simulink model "untitled9"  (R2023b)
settings: Solver=FixedStepAuto  StartTime=0.0  StopTime=2.9  FixedStep=1e-5
values from neighbouring files (symbols this model uses):
  Global_Bx = reshape(Bx, [Nx, Ny, Nz])    [init_global_map2.m]
  Global_By = reshape(By, [Nx, Ny, Nz])    [init_global_map2.m]
  Global_Bz = reshape(Bz, [Nx, Ny, Nz])    [init_global_map2.m]
  N = Nx * Ny * Nz    (= 4080501)    [init_global_map2.m]
  x_glob_range = x_glob_range(:)    [init_global_map2.m]
  y_glob_range = y_glob_range(:)    [init_global_map2.m]
  z_glob_range = z_glob_range(:)    [init_global_map2.m]
undefined symbols (not defined in the file or in its folder): X, Y, Z
libraries: sm_lib x15, nesl_utility x6, sharedtransform x2, simulink x2
settings Model: Creator=germa  LastModifiedBy=germa

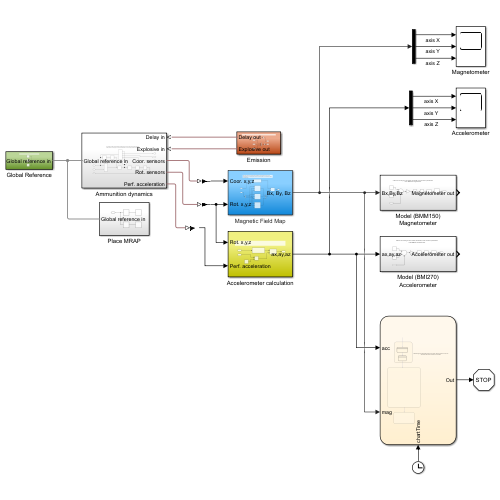
[thumbnail: Simulink's stored preview of the top-level diagram]
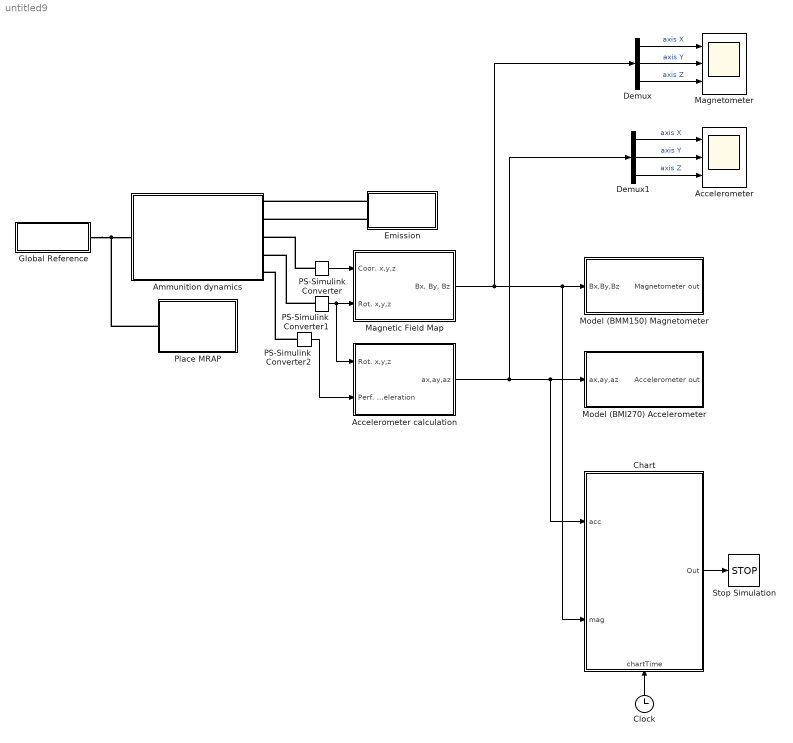
== system untitled9 ==
  Accelerometer : Scope  NumInputPorts=3
  Accelerometer calculation : Subsystem
  Ammunition dynamics : Subsystem
  Chart : Stateflow chart  TreatAsAtomicUnit=on
      settings: PortSchema="{\"entries\":[{\"content\":{\"sides\":[{\"content\":{\"connectorIds\":[\"In2\",\"In3\"]},\"type\":\"ConnectorPlacement.EquallySpacedRectSide\",\"uuid\":\"2f7f4fa5-e89a-4fc1-bed6-30d007998820\"},{\"content\":{\"connectorIds\":[\"Out1\"],\"side\":\"RIGHT\"},\"type\":\"ConnectorPlacement.EquallySpacedRectSide\",\"uuid\":\"4dcede0d-181a-4776-8973-11248acb9a50\"},{\"content\":{\"side\":\"TOP\"},\"type\":\"ConnectorPlacement.EquallySpacedRectSide\",\"uuid\":\"fd273f8e-25b4-48c5-b488-b01aba33f87d\"},{\"content\":{\"connectorIds\":[\"In1\"],\"side\":\"BOTTOM\"},\"type\":\"ConnectorPlacement.EquallySpacedRectSide\",\"uuid\":\"7dfac832-98a9-44a5-9739-cb7b49b62e5f\"}]},\"type\":\"ConnectorPlacement.EquallySpacedConnector\",\"uuid\":\"6be13ad6-9752-4a37-809e-31edad18d250\"}],\"packageUris\":[\"http://schema.mathworks.com/mf0/Connector/R2020b\"],\"version\":\"1.0\"}"
  Clock : Clock
  Demux : Demux  Outputs=3
  Demux1 : Demux  Outputs=3
  Emission : Subsystem
  Global Reference : Subsystem
  Magnetic Field Map : Subsystem
  Magnetometer : Scope  NumInputPorts=3
  Model (BMI270) Accelerometer : Subsystem
  Model (BMM150) Magnetometer : Subsystem
  PS-Simulink Converter : nesl_utility/PS-Simulink Converter  PhysicalDomain=network_engine_domain  SubClassName=ps_output  LeftPortType=input  RightPortType=output  PseudoPeriodic=off  Frequencies=[]  VectorFormat=inherit  Unit=inherit  AffineConversion=off
  PS-Simulink Converter1 : nesl_utility/PS-Simulink Converter  PhysicalDomain=network_engine_domain  SubClassName=ps_output  LeftPortType=input  RightPortType=output  PseudoPeriodic=off  Frequencies=[]  VectorFormat=inherit  Unit=inherit  AffineConversion=off
  PS-Simulink Converter2 : nesl_utility/PS-Simulink Converter  PhysicalDomain=network_engine_domain  SubClassName=ps_output  LeftPortType=input  RightPortType=output  PseudoPeriodic=off  Frequencies=[]  VectorFormat=inherit  Unit=inherit  AffineConversion=off
  Place MRAP : Subsystem
  Stop Simulation : Stop
  wires:
  PS-Simulink Converter/1 -> Magnetic Field Map/1(Coor. x,y,z)
  PS-Simulink Converter1/1 -> Accelerometer calculation/1(Rot. x,y,z), Magnetic Field Map/2(Rot. x,y,z)
  Demux/3 -> Magnetometer/3  "axis Z"
  Demux/2 -> Magnetometer/2  "axis Y"
  Demux/1 -> Magnetometer/1  "axis X"
  Magnetic Field Map/1("Bx, By, Bz") -> Demux/1, Chart/3(mag), Model (BMM150) Magnetometer/1(Bx,By,Bz)
  Demux1/3 -> Accelerometer/3  "axis Z"
  Demux1/1 -> Accelerometer/1  "axis X"
  Demux1/2 -> Accelerometer/2  "axis Y"
  PS-Simulink Converter2/1 -> Accelerometer calculation/2(Perf. acceleration)
  Accelerometer calculation/1(ax,ay,az) -> Chart/2(acc), Model (BMI270) Accelerometer/1(ax,ay,az), Demux1/1
  Clock/1 -> Chart/1(chartTime)
  Chart/1(Out) -> Stop Simulation/1
  connections:
  Emission/RConn2 -- Ammunition dynamics/RConn2
  Emission/RConn1 -- Ammunition dynamics/RConn1
  PS-Simulink Converter/LConn1 -- Ammunition dynamics/RConn3
  PS-Simulink Converter1/LConn1 -- Ammunition dynamics/RConn4
  Global Reference/LConn1 -- Place MRAP/LConn1 -- Ammunition dynamics/LConn1
  PS-Simulink Converter2/LConn1 -- Ammunition dynamics/RConn5

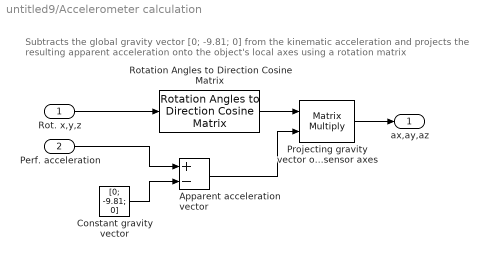
== system untitled9/Accelerometer calculation ==
  note: Subtracts the global gravity vector [0; -9.81; 0] from the kinematic acceleration and projects the resulting apparent acceleration onto the object's local axes using a rotation matrix
  Rot. x,y,z : Inport
  Perf. acceleration : Inport  Port=2
  Apparent acceleration vector : Sum  Inputs=+-
  Constant gravity vector : Constant  Value=[0; -9.81; 0]
  Projecting gravity vector onto sensor axes : Product  Multiplication=Matrix(*)
  Rotation Angles to Direction Cosine Matrix : sharedtransform/Rotation Angles to Direction Cosine Matrix  rotationOrder=XYZ  aMode=aMode
  ax,ay,az : Outport
  wires:
  Apparent acceleration vector/1 -> Projecting gravity vector onto sensor axes/2
  Perf. acceleration/1 -> Apparent acceleration vector/1
  Rot. x,y,z/1 -> Rotation Angles to Direction Cosine Matrix/1
  Rotation Angles to Direction Cosine Matrix/1 -> Projecting gravity vector onto sensor axes/1
  Constant gravity vector/1 -> Apparent acceleration vector/2
  Projecting gravity vector onto sensor axes/1 -> ax,ay,az/1

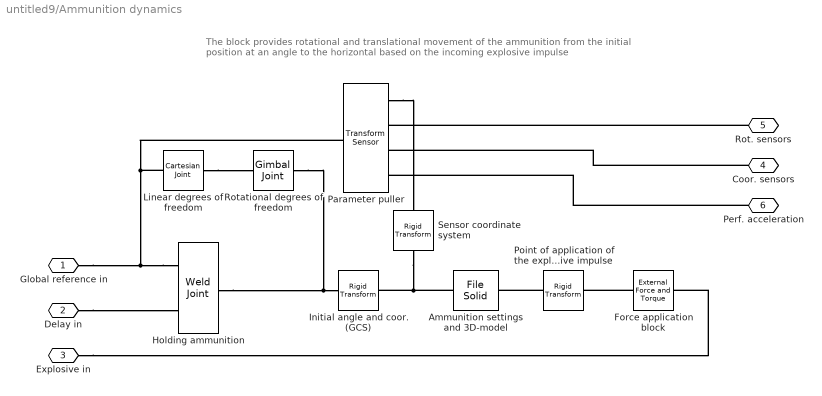
== system untitled9/Ammunition dynamics ==
  note: The block provides rotational and translational movement of the ammunition from the initial position at an angle to the horizontal based on the incoming explosive impulse
  "   Linear degrees of freedom" : sm_lib/Joints/Cartesian Joint  JointMode=Normal  SenseConstraintForce=off  SenseConstraintForceX=off  SenseConstraintForceY=off  SenseConstraintForceZ=off  SenseConstraintTorque=off  SenseConstraintTorqueX=off  SenseConstraintTorqueY=off  SenseConstraintTorqueZ=off  SenseTotalForce=off  SenseTotalForceX=off  SenseTotalForceY=off  SenseTotalForceZ=off  SenseTotalTorque=off  SenseTotalTorqueX=off  SenseTotalTorqueY=off  SenseTotalTorqueZ=off  CompositeWrenchDir=FollowerOnBase  CompositeWrenchFrame=BaseFrame  PxEquilibriumPosition=0  PxEquilibriumPositionUnits=m  PxSpringStiffness=0  PxSpringStiffnessUnits=N/m  PxDampingCoefficient=0  PxDampingCoefficientUnits=N/(m/s)  PxTorqueActuationMode=NoTorque  PxMotionActuationMode=ComputedMotion  PxSensePosition=off  PxSenseVelocity=off  PxSenseAcceleration=off  PxSenseTorqueForce=off  PxSenseLowerLimitTorqueForce=off  PxSenseUpperLimitTorqueForce=off  PxLowerLimitSpecify=off  PxLowerLimitBound=-1  PxLowerLimitBoundUnits=m  PxLowerLimitStiffness=1e6  PxLowerLimitStiffnessUnits=N/m  PxLowerLimitDamping=1e3  PxLowerLimitDampingUnits=N/(m/s)  PxLowerLimitTransitionRegionWidth=1e-4  PxLowerLimitTransitionRegionWidthUnits=m  PxUpperLimitSpecify=off  PxUpperLimitBound=1  PxUpperLimitBoundUnits=m  PxUpperLimitStiffness=1e6  PxUpperLimitStiffnessUnits=N/m  PxUpperLimitDamping=1e3  PxUpperLimitDampingUnits=N/(m/s)  PxUpperLimitTransitionRegionWidth=1e-4  PxUpperLimitTransitionRegionWidthUnits=m  PxPositionTargetSpecify=off  PxPositionTargetPriority=High  PxPositionTargetValue=0  PxPositionTargetValueUnits=m  PxVelocityTargetSpecify=off  PxVelocityTargetPriority=High  PxVelocityTargetValue=0  PxVelocityTargetValueUnits=m/s  PyEquilibriumPosition=0  PyEquilibriumPositionUnits=m  PySpringStiffness=0  PySpringStiffnessUnits=N/m  PyDampingCoefficient=0  PyDampingCoefficientUnits=N/(m/s)  PyTorqueActuationMode=NoTorque  PyMotionActuationMode=ComputedMotion  PySensePosition=off  PySenseVelocity=off  PySenseAcceleration=off  PySenseTorqueForce=off  PySenseLowerLimitTorqueForce=off  PySenseUpperLimitTorqueForce=off  PyLowerLimitSpecify=off  PyLowerLimitBound=-1  PyLowerLimitBoundUnits=m  PyLowerLimitStiffness=1e6  PyLowerLimitStiffnessUnits=N/m  PyLowerLimitDamping=1e3  PyLowerLimitDampingUnits=N/(m/s)  PyLowerLimitTransitionRegionWidth=1e-4  PyLowerLimitTransitionRegionWidthUnits=m  PyUpperLimitSpecify=off  PyUpperLimitBound=1  PyUpperLimitBoundUnits=m  PyUpperLimitStiffness=1e6  PyUpperLimitStiffnessUnits=N/m  PyUpperLimitDamping=1e3  PyUpperLimitDampingUnits=N/(m/s)  PyUpperLimitTransitionRegionWidth=1e-4  PyUpperLimitTransitionRegionWidthUnits=m  PyPositionTargetSpecify=off  PyPositionTargetPriority=High  PyPositionTargetValue=0  PyPositionTargetValueUnits=m  PyVelocityTargetSpecify=off  PyVelocityTargetPriority=High  PyVelocityTargetValue=0  PyVelocityTargetValueUnits=m/s  PzEquilibriumPosition=0  PzEquilibriumPositionUnits=m  PzSpringStiffness=0  PzSpringStiffnessUnits=N/m  PzDampingCoefficient=0  PzDampingCoefficientUnits=N/(m/s)  PzTorqueActuationMode=NoTorque  PzMotionActuationMode=ComputedMotion  PzSensePosition=off  PzSenseVelocity=off  PzSenseAcceleration=off  PzSenseTorqueForce=off  PzSenseLowerLimitTorqueForce=off  PzSenseUpperLimitTorqueForce=off  PzLowerLimitSpecify=off  PzLowerLimitBound=-1  PzLowerLimitBoundUnits=m  PzLowerLimitStiffness=1e6  PzLowerLimitStiffnessUnits=N/m  PzLowerLimitDamping=1e3  PzLowerLimitDampingUnits=N/(m/s)  PzLowerLimitTransitionRegionWidth=1e-4  PzLowerLimitTransitionRegionWidthUnits=m  PzUpperLimitSpecify=off  PzUpperLimitBound=1  PzUpperLimitBoundUnits=m  PzUpperLimitStiffness=1e6  PzUpperLimitStiffnessUnits=N/m  PzUpperLimitDamping=1e3  PzUpperLimitDampingUnits=N/(m/s)  PzUpperLimitTransitionRegionWidth=1e-4  PzUpperLimitTransitionRegionWidthUnits=m  PzPositionTargetSpecify=off  PzPositionTargetPriority=High  PzPositionTargetValue=0  PzPositionTargetValueUnits=m  PzVelocityTargetSpecify=off  PzVelocityTargetPriority=High  PzVelocityTargetValue=0  PzVelocityTargetValueUnits=m/s
  "  Rotational degrees of freedom" : sm_lib/Joints/Gimbal Joint  JointMode=Normal  SenseConstraintForce=off  SenseConstraintForceX=off  SenseConstraintForceY=off  SenseConstraintForceZ=off  SenseConstraintTorque=off  SenseConstraintTorqueX=off  SenseConstraintTorqueY=off  SenseConstraintTorqueZ=off  SenseTotalForce=off  SenseTotalForceX=off  SenseTotalForceY=off  SenseTotalForceZ=off  SenseTotalTorque=off  SenseTotalTorqueX=off  SenseTotalTorqueY=off  SenseTotalTorqueZ=off  CompositeWrenchDir=FollowerOnBase  CompositeWrenchFrame=BaseFrame  RxEquilibriumPosition=0  RxEquilibriumPositionUnits=deg  RxSpringStiffness=0  RxSpringStiffnessUnits=N*m/deg  RxDampingCoefficient=0  RxDampingCoefficientUnits=N*m/(deg/s)  RxTorqueActuationMode=NoTorque  RxMotionActuationMode=ComputedMotion  RxSensePosition=off  RxSenseVelocity=off  RxSenseAcceleration=off  RxSenseTorqueForce=off  RxSenseLowerLimitTorqueForce=off  RxSenseUpperLimitTorqueForce=off  RxLowerLimitSpecify=off  RxLowerLimitBound=-90  RxLowerLimitBoundUnits=deg  RxLowerLimitStiffness=1e4  RxLowerLimitStiffnessUnits=N*m/deg  RxLowerLimitDamping=10  RxLowerLimitDampingUnits=N*m/(deg/s)  RxLowerLimitTransitionRegionWidth=0.1  RxLowerLimitTransitionRegionWidthUnits=deg  RxUpperLimitSpecify=off  RxUpperLimitBound=90  RxUpperLimitBoundUnits=deg  RxUpperLimitStiffness=1e4  RxUpperLimitStiffnessUnits=N*m/deg  RxUpperLimitDamping=10  RxUpperLimitDampingUnits=N*m/(deg/s)  RxUpperLimitTransitionRegionWidth=0.1  RxUpperLimitTransitionRegionWidthUnits=deg  RxPositionTargetSpecify=off  RxPositionTargetPriority=High  RxPositionTargetValue=0  RxPositionTargetValueUnits=deg  RxVelocityTargetSpecify=off  RxVelocityTargetPriority=High  RxVelocityTargetValue=0  RxVelocityTargetValueUnits=deg/s  RyEquilibriumPosition=0  RyEquilibriumPositionUnits=deg  RySpringStiffness=0  RySpringStiffnessUnits=N*m/deg  RyDampingCoefficient=0  RyDampingCoefficientUnits=N*m/(deg/s)  RyTorqueActuationMode=NoTorque  RyMotionActuationMode=ComputedMotion  RySensePosition=off  RySenseVelocity=off  RySenseAcceleration=off  RySenseTorqueForce=off  RySenseLowerLimitTorqueForce=off  RySenseUpperLimitTorqueForce=off  RyLowerLimitSpecify=off  RyLowerLimitBound=-90  RyLowerLimitBoundUnits=deg  RyLowerLimitStiffness=1e4  RyLowerLimitStiffnessUnits=N*m/deg  RyLowerLimitDamping=10  RyLowerLimitDampingUnits=N*m/(deg/s)  RyLowerLimitTransitionRegionWidth=0.1  RyLowerLimitTransitionRegionWidthUnits=deg  RyUpperLimitSpecify=off  RyUpperLimitBound=90  RyUpperLimitBoundUnits=deg  RyUpperLimitStiffness=1e4  RyUpperLimitStiffnessUnits=N*m/deg  RyUpperLimitDamping=10  RyUpperLimitDampingUnits=N*m/(deg/s)  RyUpperLimitTransitionRegionWidth=0.1  RyUpperLimitTransitionRegionWidthUnits=deg  RyPositionTargetSpecify=off  RyPositionTargetPriority=High  RyPositionTargetValue=0  RyPositionTargetValueUnits=deg  RyVelocityTargetSpecify=off  RyVelocityTargetPriority=High  RyVelocityTargetValue=0  RyVelocityTargetValueUnits=deg/s  RzEquilibriumPosition=0  RzEquilibriumPositionUnits=deg  RzSpringStiffness=0  RzSpringStiffnessUnits=N*m/deg  RzDampingCoefficient=0.005  RzDampingCoefficientUnits=N*m/(deg/s)  RzTorqueActuationMode=NoTorque  RzMotionActuationMode=ComputedMotion  RzSensePosition=off  RzSenseVelocity=off  RzSenseAcceleration=off  RzSenseTorqueForce=off  RzSenseLowerLimitTorqueForce=off  RzSenseUpperLimitTorqueForce=off  RzLowerLimitSpecify=off  RzLowerLimitBound=-90  RzLowerLimitBoundUnits=deg  RzLowerLimitStiffness=1e4  RzLowerLimitStiffnessUnits=N*m/deg  RzLowerLimitDamping=10  RzLowerLimitDampingUnits=N*m/(deg/s)  RzLowerLimitTransitionRegionWidth=0.1  RzLowerLimitTransitionRegionWidthUnits=deg  RzUpperLimitSpecify=off  RzUpperLimitBound=90  RzUpperLimitBoundUnits=deg  RzUpperLimitStiffness=1e4  RzUpperLimitStiffnessUnits=N*m/deg  RzUpperLimitDamping=10  RzUpperLimitDampingUnits=N*m/(deg/s)  RzUpperLimitTransitionRegionWidth=0.1  RzUpperLimitTransitionRegionWidthUnits=deg  RzPositionTargetSpecify=off  RzPositionTargetPriority=High  RzPositionTargetValue=0  RzPositionTargetValueUnits=deg  RzVelocityTargetSpecify=off  RzVelocityTargetPriority=High  RzVelocityTargetValue=0  RzVelocityTargetValueUnits=deg/s
  Ammunition settings and 3D-model : sm_lib/Body Elements/File Solid  ExtGeomFileName=C:\Users\germa\OneDrive\Desktop\New folder\solid.stl  UnitType=Custom  ExtGeomFileUnits=mm  StepReaderType=HEX  ExportConvexHullGeometry=off  InertiaType=CalculateFromGeometry  Mass=43  MassUnits=kg  CenterOfMass=[0 0 0]  CenterOfMassUnits=m  MomentsOfInertia=[1 1 1]  MomentsOfInertiaUnits=kg*m^2  ProductsOfInertia=[0 0 0]  ProductsOfInertiaUnits=kg*m^2  BasedOnType=Mass  Density=1000  DensityUnits=kg/m^3  DoExposeReferenceFrame=on  SerializedFrames=<Frames><Frame><Id>Frame1</Id><Value><Name>Frame_Impulse</Name><Origin><Source>CenterOfMassFrame</Source><FeatureName></FeatureName></Origin><PrimaryAxis><DefinedDirection>+Z</DefinedDirection><Source>ReferenceFrame</Source><SourceDirection>+Z</SourceDirection><FeatureName></FeatureName></PrimaryAxis><SecondaryAxis><DefinedDirection>+X</DefinedDirection><Source>ReferenceFrame</Source><SourceDirection>+X</SourceDirection><FeatureName></FeatureName></SecondaryAxis></Value></Frame></Frames>  GraphicType=FromGeometry  MarkerShape=Sphere  MarkerSize=10  GraphicVisPropType=SimpleVisualProperties  GraphicDiffuseColor=[0.5 0.5 0.5]  GraphicSpecularColor=[0.5 0.5 0.5 1.0]  GraphicAmbientColor=[0.15 0.15 0.15 1.0]  GraphicEmissiveColor=[0.0 0.0 0.0 1.0]  GraphicShininess=75  GraphicOpacity=1.0
  Force application block : sm_lib/Forces and Torques/External Force and Torque  ForceResolutionFrame=AttachedFrame  EnableForceX=off  EnableForceY=off  EnableForceZ=off  EnableForce=on  TorqueResolutionFrame=AttachedFrame  EnableTorqueX=off  EnableTorqueY=off  EnableTorqueZ=off  EnableTorque=off
  Holding ammunition : sm_lib/Joints/Weld Joint  JointMode=ProvidedByInput  SenseConstraintForce=off  SenseConstraintForceX=off  SenseConstraintForceY=off  SenseConstraintForceZ=off  SenseConstraintTorque=off  SenseConstraintTorqueX=off  SenseConstraintTorqueY=off  SenseConstraintTorqueZ=off  SenseTotalForce=off  SenseTotalForceX=off  SenseTotalForceY=off  SenseTotalForceZ=off  SenseTotalTorque=off  SenseTotalTorqueX=off  SenseTotalTorqueY=off  SenseTotalTorqueZ=off  CompositeWrenchDir=FollowerOnBase  CompositeWrenchFrame=FollowerFrame
  Initial angle and coor. (GCS) : sm_lib/Frames and Transforms/Rigid Transform  TranslationMethod=Cartesian  TranslationStandardOffset=0  TranslationStandardOffsetUnits=m  TranslationStandardAxis=+Z  TranslationCartesianOffset=[10 0 25]  TranslationCartesianOffsetUnits=m  TranslationROffset=0  TranslationROffsetUnits=m  TranslationZOffset=0  TranslationZOffsetUnits=m  TranslationThetaOffset=0  TranslationThetaOffsetUnits=deg  RotationMethod=RotationSequence  RotationAngleUnits=deg  RotationStandardAxis=+Z  RotationAngle=0.0  RotationArbitraryAxis=[0 0 1]  FollAlignAxisA=+X  BaseAlignAxisA=+Y  FollAlignAxisB=+Y  BaseAlignAxisB=+Z  RotationSequenceAxes=FollowerAxes  RotationSequence=ZXY  RotationSequenceAngles=[65 1 1]  RotationSequenceAnglesUnits=deg  RotationMatrix=[1 0 0; 0 1 0; 0 0 1]  Quaternion=[1 0 0 0]
  Parameter puller : sm_lib/Frames and Transforms/Transform Sensor  MeasurementFrame=World  RotationSequence=XYZ  SenseAngle=off  SenseAxis=off  SenseQ=off  SenseR=off  SenseRotationSequence=on  SenseOmegaX=off  SenseOmegaY=off  SenseOmegaZ=off  SenseOmega=off  SenseQDot=off  SenseRDot=off  SenseRotationSequenceDot=off  SenseAlphaX=off  SenseAlphaY=off  SenseAlphaZ=off  SenseAlpha=off  SenseQDDot=off  SenseRDDot=off  SenseX=off  SenseY=off  SenseZ=off  SenseXYZ=on  SenseRad=off  SenseAzim=off  SenseDist=off  SenseInc=off  SenseXDot=off  SenseYDot=off  SenseZDot=off  SenseXYZDot=off  SenseRadDot=off  SenseAzimDot=off  SenseDistDot=off  SenseIncDot=off  SenseXDDot=off  SenseYDDot=off  SenseZDDot=off  SenseXYZDDot=on  SenseRadDDot=off  SenseAzimDDot=off  SenseDistDDot=off  SenseIncDDot=off
  Point of application of the explosive impulse : sm_lib/Frames and Transforms/Rigid Transform  TranslationMethod=Cartesian  TranslationStandardOffset=0  TranslationStandardOffsetUnits=m  TranslationStandardAxis=+Z  TranslationCartesianOffset=[10 95 3]  TranslationCartesianOffsetUnits=mm  TranslationROffset=0  TranslationROffsetUnits=m  TranslationZOffset=0  TranslationZOffsetUnits=m  TranslationThetaOffset=0  TranslationThetaOffsetUnits=deg  RotationMethod=None  RotationAngleUnits=deg  RotationStandardAxis=+Z  RotationAngle=0.0  RotationArbitraryAxis=[0 0 1]  FollAlignAxisA=+X  BaseAlignAxisA=+Y  FollAlignAxisB=+Y  BaseAlignAxisB=+Z  RotationSequenceAxes=FollowerAxes  RotationSequence=XYX  RotationSequenceAngles=[0 0 0]  RotationSequenceAnglesUnits=deg  RotationMatrix=[1 0 0; 0 1 0; 0 0 1]  Quaternion=[1 0 0 0]
  Sensor coordinate system : sm_lib/Frames and Transforms/Rigid Transform  TranslationMethod=Cartesian  TranslationStandardOffset=0  TranslationStandardOffsetUnits=m  TranslationStandardAxis=+Z  TranslationCartesianOffset=[0 417 0]  TranslationCartesianOffsetUnits=mm  TranslationROffset=0  TranslationROffsetUnits=m  TranslationZOffset=0  TranslationZOffsetUnits=m  TranslationThetaOffset=0  TranslationThetaOffsetUnits=deg  RotationMethod=None  RotationAngleUnits=deg  RotationStandardAxis=+Z  RotationAngle=0.0  RotationArbitraryAxis=[0 0 1]  FollAlignAxisA=+X  BaseAlignAxisA=+Y  FollAlignAxisB=+Y  BaseAlignAxisB=+Z  RotationSequenceAxes=FollowerAxes  RotationSequence=XYX  RotationSequenceAngles=[0 0 0]  RotationSequenceAnglesUnits=deg  RotationMatrix=[1 0 0; 0 1 0; 0 0 1]  Quaternion=[1 0 0 0]
  Global reference in : PMIOPort  Side=Left
  Delay in : PMIOPort  Port=2  Side=Right
  Explosive in : PMIOPort  Port=3  Side=Right
  Coor. sensors : PMIOPort  Port=4  Side=Right
  Rot. sensors : PMIOPort  Port=5  Side=Right
  Perf. acceleration : PMIOPort  Port=6  Side=Right
  connections:
  "  Rotational degrees of freedom"/RConn1 -- Holding ammunition/RConn1 -- Initial angle and coor. (GCS)/LConn1
  Holding ammunition/LConn1 -- Parameter puller/LConn1 -- "   Linear degrees of freedom"/LConn1 -- Global reference in/RConn1
  "   Linear degrees of freedom"/RConn1 -- "  Rotational degrees of freedom"/LConn1
  Force application block/RConn1 -- Point of application of the explosive impulse/RConn1
  Sensor coordinate system/LConn1 -- Ammunition settings and 3D-model/RConn1 -- Initial angle and coor. (GCS)/RConn1
  Parameter puller/RConn1 -- Sensor coordinate system/RConn1
  Delay in/RConn1 -- Holding ammunition/LConn2
  Point of application of the explosive impulse/LConn1 -- Ammunition settings and 3D-model/LConn1
  Explosive in/RConn1 -- Force application block/LConn1
  Rot. sensors/RConn1 -- Parameter puller/RConn2
  Coor. sensors/RConn1 -- Parameter puller/RConn3
  Perf. acceleration/RConn1 -- Parameter puller/RConn4

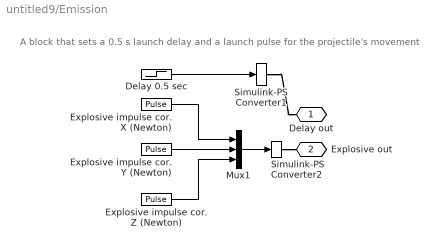
== system untitled9/Emission ==
  note: A block that sets a 0.5 s launch delay and a launch pulse for the projectile's movement
  Delay 0.5 sec : Step  Time=0.5  After=-1  SampleTime=0.001
  Explosive impulse cor. X (Newton) : DiscretePulseGenerator  PulseType=Time based  Amplitude=12000  Period=50  PulseWidth=0.1  PhaseDelay=0.5
  Explosive impulse cor. Y (Newton) : DiscretePulseGenerator  PulseType=Time based  Amplitude=5000  Period=50  PulseWidth=0.1  PhaseDelay=0.5
  Explosive impulse cor. Z (Newton) : DiscretePulseGenerator  PulseType=Time based  Amplitude=-150  Period=50  PulseWidth=0.1  PhaseDelay=0.5
  Mux1 : Mux  Inputs=3
  Simulink-PS Converter1 : nesl_utility/Simulink-PS Converter  PhysicalDomain=network_engine_domain  SubClassName=ps_input  LeftPortType=input  RightPortType=output  PseudoPeriodic=off  Frequencies=[]  NoiseDistribution=none  NoiseParameters=[]  Unit=1  AffineConversion=off  FilteringAndDerivatives=provide  SimscapeFilterOrder=1  InputFilterTimeConstant=0.001  UdotUserProvided=0
  Simulink-PS Converter2 : nesl_utility/Simulink-PS Converter  PhysicalDomain=network_engine_domain  SubClassName=ps_input  LeftPortType=input  RightPortType=output  PseudoPeriodic=off  Frequencies=[]  NoiseDistribution=none  NoiseParameters=[]  Unit=N  AffineConversion=off  FilteringAndDerivatives=provide  SimscapeFilterOrder=1  InputFilterTimeConstant=0.001  UdotUserProvided=0
  Delay out : PMIOPort  Side=Right
  Explosive out : PMIOPort  Port=2  Side=Right
  wires:
  Explosive impulse cor. X (Newton)/1 -> Mux1/1
  Explosive impulse cor. Y (Newton)/1 -> Mux1/2
  Mux1/1 -> Simulink-PS Converter2/1
  Explosive impulse cor. Z (Newton)/1 -> Mux1/3
  Delay 0.5 sec/1 -> Simulink-PS Converter1/1
  connections:
  Simulink-PS Converter1/RConn1 -- Delay out/RConn1
  Simulink-PS Converter2/RConn1 -- Explosive out/RConn1

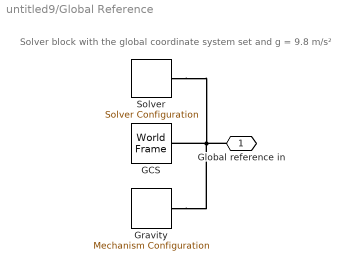
== system untitled9/Global Reference ==
  note: Solver block with the global coordinate system set and g = 9.8 m/s²
  GCS : sm_lib/Frames and Transforms/World Frame
  Gravity : sm_lib/Utilities/Mechanism Configuration  UniformGravity=Constant  GravityVector=[0 -9.81 0]  GravityVectorUnits=m/s^2  LinearizationDelta=0.001  JointModeTransitionNonlinearIterations=50
  Solver : nesl_utility/Solver Configuration  PhysicalDomain=network_engine_domain  SubClassName=solver  LeftPortType=input  RightPortType=generic  Tones=[]  Harmonics=[]  SimulateNoise=off  Profile=off  UseLocalSampling=off  EnableSwitchedLinearOptims=on  FrequencyDomain=off  UseCCode=off  RelTol=0.001  AbsTol=1e-06  MinStep=1e-09  ToWorkspace=off  RevertToSquareIcSolve=off  NumHomotopyIterations=100  PhasorMode=off  PhasorModeNumHarmonics=1  ConsistencySolver=NEWTON_XTOL_AFTER_FTOL  IndexReductionMethod=DerivativeReplacement  DoDC=off  ResidualTolerance=1e-09  ConsistencyTolSource=GLOBAL  ConsistencyAbsTol=0.001  ConsistencyRelTol=0.001  ConsistencyTolFactor=0.001  UseLocalSolver=off  LocalSolverChoice=NE_BACKWARD_EULER_ADVANCER  ResolveIndetEquations=on  FunctionEvalNumThread=1  LocalSolverSampleTime=0.001  DoFixedCost=off  MaxNonlinIter=3  MaxModeIter=2  ComputeImpulses=off  ImpulseIterations=2  LinearAlgebra=Sparse  LinearAlgebraNumThread=0  EquationFormulation=NE_TIME_EF  DelaysMemoryBudget=1024  AutomaticFiltering=on  FilteringTimeConstant=0.001  PartitionStorageMethod=AS_NEEDED  PartitionMemoryBudget=1024  PartitionMethod=FAST  MultibodyUseLocalSolver=off  MultibodyLocalSolverChoice=ODE1  MultibodyLocalSolverSampleTime=0.001
  Global reference in : PMIOPort  Side=Left
  connections:
  Global reference in/RConn1 -- Gravity/RConn1 -- Solver/RConn1 -- GCS/RConn1

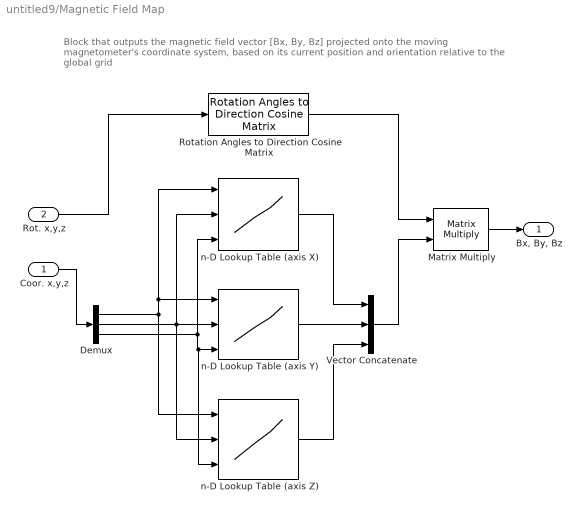
== system untitled9/Magnetic Field Map ==
  note: Block that outputs the magnetic field vector [Bx, By, Bz] projected onto the moving magnetometer's coordinate system, based on its current position and orientation relative to the global grid
  Coor. x,y,z : Inport
  Rot. x,y,z : Inport  Port=2
  Demux : Demux  Outputs=3
  Matrix Multiply : Product  Multiplication=Matrix(*)
  Rotation Angles to Direction Cosine Matrix : sharedtransform/Rotation Angles to Direction Cosine Matrix  rotationOrder=XYZ  aMode=aMode
  Vector Concatenate : Concatenate  NumInputs=3  Mode=Multidimensional array
  n-D Lookup Table (axis X) : Lookup_n-D  NumberOfTableDimensions=3  BreakpointsForDimension1=x_glob_range  BreakpointsForDimension2=y_glob_range  BreakpointsForDimension3=z_glob_range  BreakpointsForDimension4=[1]  Table=Global_Bx  InternalRulePriority=Speed  RndMeth=Simplest
      settings: InputPortMap=u0,u1,u2
  n-D Lookup Table (axis Y) : Lookup_n-D  NumberOfTableDimensions=3  BreakpointsForDimension1=x_glob_range  BreakpointsForDimension2=y_glob_range  BreakpointsForDimension3=z_glob_range  BreakpointsForDimension4=[1]  Table=Global_By  InternalRulePriority=Speed  RndMeth=Simplest
      settings: InputPortMap=u0,u1,u2
  n-D Lookup Table (axis Z) : Lookup_n-D  NumberOfTableDimensions=3  BreakpointsForDimension1=x_glob_range  BreakpointsForDimension2=y_glob_range  BreakpointsForDimension3=z_glob_range  BreakpointsForDimension4=[1]  Table=Global_Bz  InternalRulePriority=Speed  RndMeth=Simplest
      settings: InputPortMap=u0,u1,u2
  "Bx, By, Bz" : Outport
  wires:
  Coor. x,y,z/1 -> Demux/1
  n-D Lookup Table (axis Z)/1 -> Vector Concatenate/3
  n-D Lookup Table (axis Y)/1 -> Vector Concatenate/2
  Demux/2 -> n-D Lookup Table (axis Z)/2, n-D Lookup Table (axis X)/2, n-D Lookup Table (axis Y)/2
  Demux/1 -> n-D Lookup Table (axis Y)/1, n-D Lookup Table (axis X)/1, n-D Lookup Table (axis Z)/1
  n-D Lookup Table (axis X)/1 -> Vector Concatenate/1
  Demux/3 -> n-D Lookup Table (axis X)/3, n-D Lookup Table (axis Z)/3, n-D Lookup Table (axis Y)/3
  Rot. x,y,z/1 -> Rotation Angles to Direction Cosine Matrix/1
  Matrix Multiply/1 -> "Bx, By, Bz"/1
  Vector Concatenate/1 -> Matrix Multiply/2
  Rotation Angles to Direction Cosine Matrix/1 -> Matrix Multiply/1

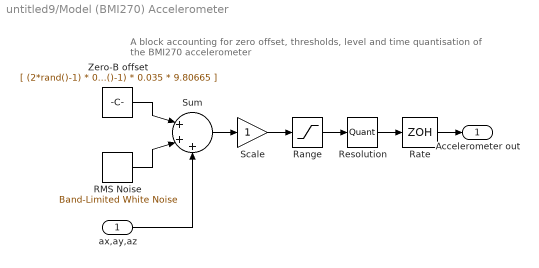
== system untitled9/Model (BMI270) Accelerometer ==
  note: A block accounting for zero offset, thresholds, level and time quantisation
      | of the BMI270 accelerometer
  ax,ay,az : Inport
  RMS Noise : simulink/Sources/Band-Limited White Noise  Cov=[2e-8; 2e-8; 2e-8]  Ts=1e-5  seed=[23341]  VectorParams1D=off
  Range : Saturate  UpperLimit=[19.613; 19.613; 19.613]  LowerLimit=[-1300e-6; -1300e-6; -2500e-6]
  Rate : ZeroOrderHold  SampleTime=0.01
  Resolution : Quantizer  QuantizationInterval=[0.0005985; 0.0005985; 0.0005985]  LinearizeAsGain=off
  Scale : Gain
  Sum : Sum  Inputs=|+++
  Zero-B offset : Constant  Value="[ (2*rand()-1) * 0.020 * 9.80665;  (2*rand()-1) * 0.020 * 9.80665;  (2*rand()-1) * 0.035 * 9.80665 ]"  VectorParams1D=off
  Accelerometer out : Outport
  wires:
  ax,ay,az/1 -> Sum/3
  RMS Noise/1 -> Sum/2
  Zero-B offset/1 -> Sum/1
  Sum/1 -> Scale/1
  Range/1 -> Resolution/1
  Resolution/1 -> Rate/1
  Rate/1 -> Accelerometer out/1
  Scale/1 -> Range/1

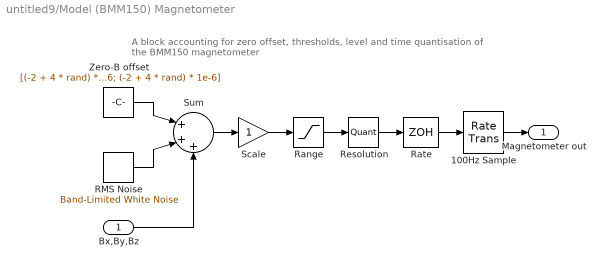
== system untitled9/Model (BMM150) Magnetometer ==
  note: A block accounting for zero offset, thresholds, level and time quantisation
      | of the BMM150 magnetometer
  Bx,By,Bz : Inport
  100Hz Sample : RateTransition  Deterministic=off  OutPortSampleTime=1/100
  RMS Noise : simulink/Sources/Band-Limited White Noise  Cov=[(0.4e-6)^2 * 1e-5; (0.4e-6)^2 * 1e-5; (0.4e-6)^2 * 1e-5]  Ts=1e-5  seed=[23341]  VectorParams1D=off
  Range : Saturate  UpperLimit=[1300e-6; 1300e-6; 2500e-6]  LowerLimit=[-1300e-6; -1300e-6; -2500e-6]
  Rate : ZeroOrderHold  SampleTime=0.01667
  Resolution : Quantizer  QuantizationInterval=0.3e-6  LinearizeAsGain=off
  Scale : Gain
  Sum : Sum  Inputs=|+++
  Zero-B offset : Constant  Value=[(-2 + 4 * rand) * 1e-6; (-2 + 4 * rand) * 1e-6; (-2 + 4 * rand) * 1e-6]  VectorParams1D=off
  Magnetometer out : Outport
  wires:
  Bx,By,Bz/1 -> Sum/3
  RMS Noise/1 -> Sum/2
  Zero-B offset/1 -> Sum/1
  Sum/1 -> Scale/1
  Range/1 -> Resolution/1
  Resolution/1 -> Rate/1
  Rate/1 -> 100Hz Sample/1
  Scale/1 -> Range/1
  100Hz Sample/1 -> Magnetometer out/1

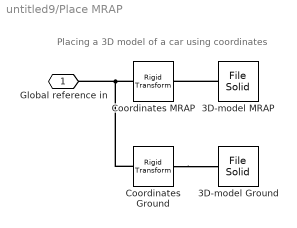
== system untitled9/Place MRAP ==
  note: Placing a 3D model of a car using coordinates
  3D-model Ground : sm_lib/Body Elements/File Solid  ExtGeomFileName=C:\Users\germa\OneDrive\Desktop\New folder\ground.stp  UnitType=Custom  ExtGeomFileUnits=mm  StepReaderType=HEX  ExportConvexHullGeometry=off  InertiaType=PointMass  Mass=0  MassUnits=kg  CenterOfMass=[0 0 0]  CenterOfMassUnits=m  MomentsOfInertia=[1 1 1]  MomentsOfInertiaUnits=kg*m^2  ProductsOfInertia=[0 0 0]  ProductsOfInertiaUnits=kg*m^2  BasedOnType=Mass  Density=1000  DensityUnits=kg/m^3  DoExposeReferenceFrame=on  SerializedFrames=<Frames/>  GraphicType=FromGeometry  MarkerShape=Sphere  MarkerSize=10  GraphicVisPropType=FromFileVisualProperties  GraphicDiffuseColor=[0.5 0.5 0.5]  GraphicSpecularColor=[0.5 0.5 0.5 1.0]  GraphicAmbientColor=[0.15 0.15 0.15 1.0]  GraphicEmissiveColor=[0.0 0.0 0.0 1.0]  GraphicShininess=75  GraphicOpacity=1.0
  3D-model MRAP : sm_lib/Body Elements/File Solid  ExtGeomFileName=C:\Users\germa\OneDrive\Desktop\New folder\MRAP.stp  UnitType=Custom  ExtGeomFileUnits=mm  StepReaderType=HEX  ExportConvexHullGeometry=off  InertiaType=PointMass  Mass=0  MassUnits=kg  CenterOfMass=[0 0 0]  CenterOfMassUnits=m  MomentsOfInertia=[1 1 1]  MomentsOfInertiaUnits=kg*m^2  ProductsOfInertia=[0 0 0]  ProductsOfInertiaUnits=kg*m^2  BasedOnType=Mass  Density=1000  DensityUnits=kg/m^3  DoExposeReferenceFrame=on  SerializedFrames=<Frames/>  GraphicType=FromGeometry  MarkerShape=Sphere  MarkerSize=10  GraphicVisPropType=SimpleVisualProperties  GraphicDiffuseColor=[0.5 0.5 0.5]  GraphicSpecularColor=[0.5 0.5 0.5 1.0]  GraphicAmbientColor=[0.15 0.15 0.15 1.0]  GraphicEmissiveColor=[0.0 0.0 0.0 1.0]  GraphicShininess=75  GraphicOpacity=1.0
  Coordinates Ground : sm_lib/Frames and Transforms/Rigid Transform  TranslationMethod=Cartesian  TranslationStandardOffset=10  TranslationStandardOffsetUnits=m  TranslationStandardAxis=+X  TranslationCartesianOffset=[0 0 0]  TranslationCartesianOffsetUnits=m  TranslationROffset=0  TranslationROffsetUnits=m  TranslationZOffset=0  TranslationZOffsetUnits=m  TranslationThetaOffset=0  TranslationThetaOffsetUnits=deg  RotationMethod=None  RotationAngleUnits=deg  RotationStandardAxis=+Z  RotationAngle=0.0  RotationArbitraryAxis=[0 0 1]  FollAlignAxisA=+X  BaseAlignAxisA=+Y  FollAlignAxisB=+Y  BaseAlignAxisB=+Z  RotationSequenceAxes=FollowerAxes  RotationSequence=XYX  RotationSequenceAngles=[0 0 0]  RotationSequenceAnglesUnits=deg  RotationMatrix=[1 0 0; 0 1 0; 0 0 1]  Quaternion=[1 0 0 0]
  Coordinates MRAP : sm_lib/Frames and Transforms/Rigid Transform  TranslationMethod=Cartesian  TranslationStandardOffset=10  TranslationStandardOffsetUnits=m  TranslationStandardAxis=+X  TranslationCartesianOffset=[20 1.78 20]  TranslationCartesianOffsetUnits=m  TranslationROffset=0  TranslationROffsetUnits=m  TranslationZOffset=0  TranslationZOffsetUnits=m  TranslationThetaOffset=0  TranslationThetaOffsetUnits=deg  RotationMethod=None  RotationAngleUnits=deg  RotationStandardAxis=+Z  RotationAngle=0.0  RotationArbitraryAxis=[0 0 1]  FollAlignAxisA=+X  BaseAlignAxisA=+Y  FollAlignAxisB=+Y  BaseAlignAxisB=+Z  RotationSequenceAxes=FollowerAxes  RotationSequence=XYX  RotationSequenceAngles=[0 0 0]  RotationSequenceAnglesUnits=deg  RotationMatrix=[1 0 0; 0 1 0; 0 0 1]  Quaternion=[1 0 0 0]
  Global reference in : PMIOPort  Side=Left
  connections:
  Coordinates MRAP/LConn1 -- Coordinates Ground/LConn1 -- Global reference in/RConn1
  3D-model MRAP/RConn1 -- Coordinates MRAP/RConn1
  Coordinates Ground/RConn1 -- 3D-model Ground/RConn1

== stateflow chart untitled9/Chart ==
  state CALC_Calibration
    state Average
      state Accumulate
        during:
        acc_sum = acc_sum + acc;
        mag_sum = mag_sum + mag;
        idx = idx + 1;
      state Compute
        during:
        mean_acc = acc_sum / idx;
        mean_mag = mag_sum / idx;
        B_static = norm(mean_mag);
        threshold = B_static * 1.03;
      note: Calculation of the average value
          | across all axes and the magnetic
          | field magnitude threshold
      (default) -> Accumulate
      Accumulate -> Compute : [idx >= 20]
    state Delay
      state Normal
        entry:
        const_acc = abs(mean_acc(2));
        during:
        cos_g_Y = abs(mean_acc(2)) / norm(mean_acc);
        cos_g_Y = max(0.0, min(1.0, cos_g_Y));
        angle_g_Y = acosd(cos_g_Y);
        cos_B_Y = abs(mean_mag(2)) / norm(mean_mag);
        cos_B_Y = max(0.0, min(1.0, cos_B_Y));
        angle_B_Y = acosd(cos_B_Y);
        angle_phase = angle_B_Y - angle_g_Y;
        if angle_phase > 90
        angle_phase = angle_phase - 180;
        elseif angle_phase < -90
        angle_phase = angle_phase + 180;
        end
      note: Based on the saved average vector values, it calculates the tilt angles of the gravity and geomagnetic field vectors relative to the sensor's Y-axis. It computes the constant difference between these angles (phase shift) and adjusts it to an invariant range from -90 to +90 degrees, avoiding the effect of the sensor being flipped 180 degrees. The resulting angle is then used as a reference for aligning the measurement zero with the horizon.
      (default) -> Normal
    Average -> Delay : [after(250, msec)]
  note: Determining the initial static state of the system, filtering sensor noise, and calculating the basic geometry of the fields.
  state CALC_Time_Shift
    entry:
    prev_signal = mag(2);
    t_zero_previous = chartTime;
    peak_count = 0;
    during:
    signal = mag(2);
    current_time = chartTime;
    % 1. Ловим пересечение нуля (смена знака синусоиды)
    if (prev_signal * signal) <= 0.0
    t_zero_current = current_time;
    if peak_count == 0
    t_zero_previous = t_zero_current;
    peak_count = 1;
    else
    % Расстояние между двумя нулями — это ПОЛУПЕРИОД
    half_period = t_zero_current - t_zero_previous;
    if half_period > 0
    % Вычисляем временной сдвиг
    time_shift = (angle_phase / 180.0) * half_period;
    t_aligned = t_zero_current - time_shift;
    mag_norm = norm(mag);
    if mag_norm > threshold
    threshold_triggered = true;
    end
    end
    t_zero_previous = t_zero_current;
    peak_count = peak_count + 1;
    end
    end
    prev_signal = signal;
  state WAIT_Aligned_Time
    entry:
    Out = false;
    t_predicted = t_aligned + half_period;
    during:
    if chartTime >= t_predicted
    Out = true;
    end
  (default) -> Average
  Delay -> CALC_Time_Shift : [abs(abs(acc(2)) - const_acc) > 0.1]
  CALC_Time_Shift -> WAIT_Aligned_Time : [threshold_triggered]
  data: chartTime input size=1; acc input size=[3 1]; mag input size=[3 1]; acc_sum local size=[3 1] =[0; 0; 0]; mag_sum local size=[3 1] =[0; 0; 0]; idx local size=1 =0; cos_g_Y local size=1 =0; cos_B_Y local size=1 =0; angle_g_Y local size=1 =0; angle_B_Y local size=1 =0; angle_phase local size=1 =0; const_acc local size=1 =0; current_time local size=1 =0; peak_count local size=1 =0; prev_signal local size=1 =0; signal local size=1 =0; half_period local size=1 =0; t_aligned local size=1 =0; t_zero_previous local size=1 =0; t_zero_current local size=1 =0; threshold local size=1 =0; B_static local size=1 =0; threshold_triggered local boolean size=1 =false; Out output =false; time_shift local size=1 =0; mean_mag local size=[3 1] =0; mean_acc local size=[3 1] =0; mag_norm local size=1 =0; t_predicted local size=[1 1] =0
